simulink model "homework2_1"  (R2023a)
settings: Solver=VariableStepAuto  StartTime=0.0  StopTime=0.5  RelTol=1e-3
undefined symbols (not defined in the file): D1, lagging, pulse
libraries: spsMultimeterLib x4, spsPLL3phLib x1, spsPulseGeneratorThyristor6PulseLib x1, spsSeriesRLCBranchLib x1, spsThreePhaseVIMeasurementLib x1, spsThreePhaseSourceLib x1, spsUniversalBridgeLib x1, sps_lib x1
settings Model: Creator=zou20  LastModifiedBy=zou20

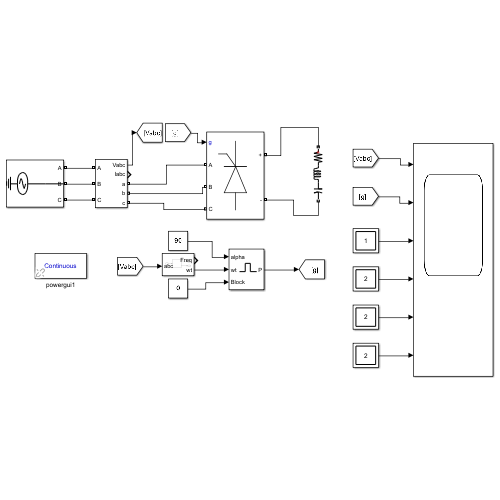
[thumbnail: Simulink's stored preview of the top-level diagram]
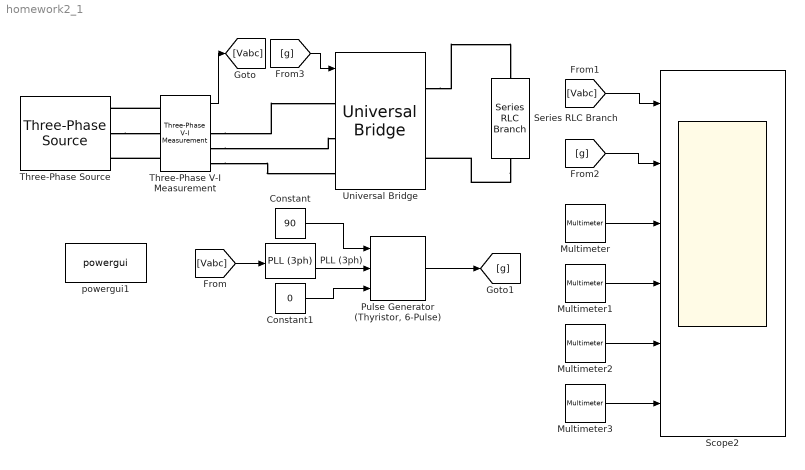
== system homework2_1 ==
  Constant : Constant  Value=90
  Constant1 : Constant  Value=0
  Multimeter : spsMultimeterLib/Multimeter  L=18  sel=1  yselected={}  Gain=1  OutputType=Complex  PlotAtSimulationStop=off  PhasorSimulation=off
  Multimeter1 : spsMultimeterLib/Multimeter  L=18  sel=[2 13]  yselected={}  Gain=[1 1]  OutputType=Complex  PlotAtSimulationStop=off  PhasorSimulation=off
  Multimeter2 : spsMultimeterLib/Multimeter  L=18  sel=[3 14]  yselected={}  Gain=[1 1]  OutputType=Complex  PlotAtSimulationStop=off  PhasorSimulation=off
  Multimeter3 : spsMultimeterLib/Multimeter  L=18  sel=[5 16]  yselected={}  Gain=[1 1]  OutputType=Complex  PlotAtSimulationStop=off  PhasorSimulation=off
  PLL (3ph) : spsPLL3phLib/PLL (3ph)  Fmin=45  Par_Init=[0, 50]  ParK=[180, 3200, 1]  TcD=1e-4  MaxRateChangeFreq=12  FilterCutOffFreq=25  Ts=0  AGC=on
  "Pulse Generator (Thyristor, 6-Pulse)" : spsPulseGeneratorThyristor6PulseLib/Pulse Generator (Thyristor, 6-Pulse)  GenType=6-pulse  Delta=D1 (lagging)  pwidth=80  Double_Pulse=off  Ts=0
      settings: LibrarySourceBlock=|
      | sps_lib/Power Electronics/Power Electronics Control/Pulse Generator
      | (Thyristor, 6-Pulse)
  Scope2 : Scope  NumInputPorts=6
  Series RLC Branch : spsSeriesRLCBranchLib/Series RLC Branch  LConnTagsString=__new0  RConnTagsString=__new0  BranchType=RLC  Resistance=1  Inductance=0  SetiL0=off  InitialCurrent=0  Capacitance=0  Setx0=off  InitialVoltage=0  Measurements=Branch voltage and current
  Three-Phase V-I Measurement : spsThreePhaseVIMeasurementLib/Three-Phase V-I Measurement  VoltageMeasurement=phase-to-ground  SetLabelV=off  LabelV=Vabc  Vpu=off  VpuLL=off  CurrentMeasurement=yes  SetLabelI=off  LabelI=Iabc  Ipu=off  Pbase=100e6  Vbase=500e3  OutputType=Complex  PhasorSimulation=off  PSBequivalent=0
  Three-Phase Source : spsThreePhaseSourceLib/Three-Phase Source  InternalConnection=Yg  VoltagePhases=off  Voltage=25e3  PhaseAngle=0  Voltage_phases=[25e3 25e3 25e3]/sqrt(3)  PhaseAngles_phases=[0 -120 +120]  Frequency=50  NonIdealSource=off  SpecifyImpedance=off  Resistance=0.8929  Inductance=16.58e-3  ShortCircuitLevel=100e6  BaseVoltage=25e3  XRratio=7  BusType=swing  Pref=10e3  Qref=0  Prefabc=[10e3, 10e3, 10e3]  Qrefabc=[0, 0, 0]  Qmin=-inf  Qmax=inf
  Universal Bridge : spsUniversalBridgeLib/Universal Bridge  Arms=3  SnubberResistance=1e5  SnubberCapacitance=inf  Device=Thyristors  Ron=1e-3  Lon=0  ForwardVoltages="[  0  0  ]"  ForwardVoltage=0  GTOparameters=[ 10e-6 , 20e-6 ]  IGBTparameters=[ 1e-6 , 2e-6 ]  Measurements=All voltages and currents  Measurements_2=None  converterType=Rectifier
  powergui1 : sps_lib/powergui  Priority=1  SimulationMode=Continuous  SampleTime=50e-6  frequency=60  Iterations=50  frequencyindice=50  Pbase=100e6  ErrMax=1e-4  UnitsV=kV  UnitsW=MW  buscounter=0  FunctionMessages=off  echomessages=off  EnableUseOfTLC=off  CurrentSourceSwitches=off  DisableSnubberDevices=off  DisableRonSwitches=off  DisableVfSwitches=off  DisplayEquations=off  AutomaticDiscreteSolvers=off  SolverType=Tustin/Backward Euler (TBE)  Interpol=off  ExternalGateDelay=off  methode=off  Ts=100  x0status=blocks  SPID=on  SwTol=0  HookPort=off  NonlinearTolerance=1e-4  nMaxIteration=100  ContinueOnMaxIteration=off  RestoreLinks=warning  ResistiveCurrentMeasurement=off  Frange=[0:2:500]  Ylog=off  Xlog=on  ShowGrid=off  save=off  variable=ZData  structure=0  ZoomFFT=off  StartTime=0.0  cycles=1  DisplayStyle=1  fundamental=60  FreqAxis=off  MaxFrequency=1000  frequencyindicesteady=1  RmsSteady=1  display=off
  wires:
  Three-Phase V-I Measurement/1 -> [Vabc]
  [Vabc] -> PLL (3ph)/1
  PLL (3ph)/2 -> "Pulse Generator (Thyristor, 6-Pulse)"/2
  Constant/1 -> "Pulse Generator (Thyristor, 6-Pulse)"/1
  Constant1/1 -> "Pulse Generator (Thyristor, 6-Pulse)"/3
  "Pulse Generator (Thyristor, 6-Pulse)"/1 -> [g]
  [Vabc] -> Scope2/1
  [g] -> Scope2/2
  [g] -> Universal Bridge/1
  Multimeter/1 -> Scope2/3
  Multimeter1/1 -> Scope2/4
  Multimeter2/1 -> Scope2/5
  Multimeter3/1 -> Scope2/6
  connections:
  Three-Phase V-I Measurement/LConn1 -- Three-Phase Source/RConn1
  Three-Phase Source/RConn2 -- Three-Phase V-I Measurement/LConn2
  Three-Phase V-I Measurement/LConn3 -- Three-Phase Source/RConn3
  Three-Phase V-I Measurement/RConn1 -- Universal Bridge/LConn1
  Three-Phase V-I Measurement/RConn2 -- Universal Bridge/LConn2
  Three-Phase V-I Measurement/RConn3 -- Universal Bridge/LConn3
  Universal Bridge/RConn1 -- Series RLC Branch/LConn1
  Series RLC Branch/RConn1 -- Universal Bridge/RConn2
